simulink model "Block_PI_regulator"  (R2022a)
settings: Solver=ode23tb  StartTime=0.0  StopTime=6  MaxStep=1e4  RelTol=1e-5
undefined symbols (not defined in the file): DiscIntNeverNeededParam, PI_reg
settings Model: Creator=админ  LastModifiedBy=админ

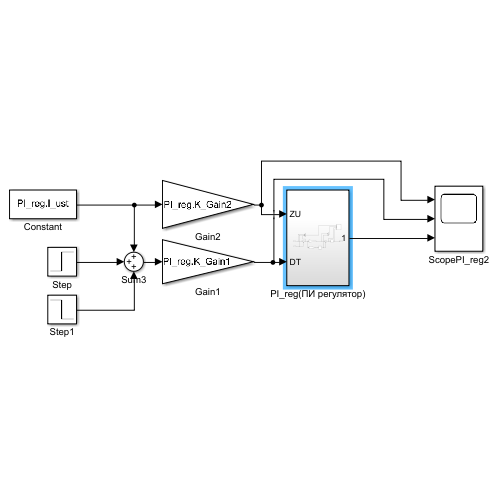
[thumbnail: Simulink's stored preview of the top-level diagram]
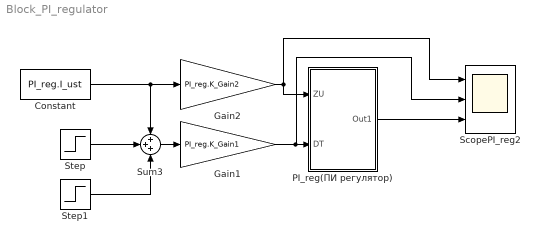
== system Block_PI_regulator ==
  Constant : Constant  Value=PI_reg.I_ust
  Gain1 : Gain  Gain=PI_reg.K_Gain1
  Gain2 : Gain  Gain=PI_reg.K_Gain2
  PI_reg(ПИ регулятор) : Subsystem
  ScopePI_reg2 : Scope  NumInputPorts=3
  Step : Step  Time=PI_reg.Step_time  After=PI_reg.Step_FinalValue  SampleTime=0
  Step1 : Step  Time=PI_reg.Step1_time  After=PI_reg.Step1_FinalValue  SampleTime=0
  Sum3 : Sum  Inputs=+++
  wires:
  Sum3/1 -> Gain1/1
  Gain1/1 -> ScopePI_reg2/2, PI_reg(ПИ регулятор)/2(DT)
  Gain2/1 -> PI_reg(ПИ регулятор)/1(ZU), ScopePI_reg2/1
  Constant/1 -> Sum3/1, Gain2/1
  Step/1 -> Sum3/2
  Step1/1 -> Sum3/3
  PI_reg(ПИ регулятор)/1(Out1) -> ScopePI_reg2/3

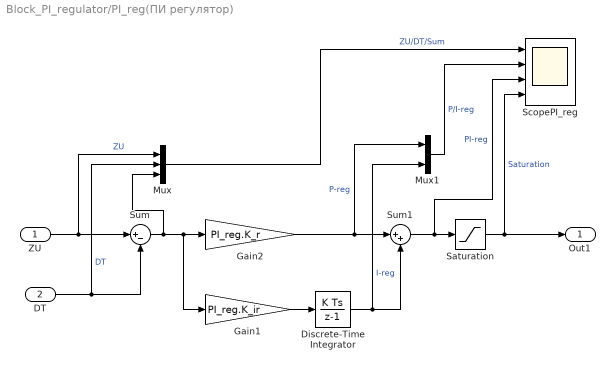
== system Block_PI_regulator/PI_reg(ПИ регулятор) ==
  ZU : Inport
  DT : Inport  Port=2
  Discrete-Time Integrator : DiscreteIntegrator  SampleTime=PI_reg.DTI_st  ICPrevOutput=DiscIntNeverNeededParam  ICPrevScaledInput=DiscIntNeverNeededParam
  Gain1 : Gain  Gain=PI_reg.K_ir
  Gain2 : Gain  Gain=PI_reg.K_r
  Mux : Mux  Inputs=3
  Mux1 : Mux  Inputs=2
  Saturation : Saturate  UpperLimit=PI_reg.StUp_limit  LowerLimit=PI_reg.StLow_limit
  ScopePI_reg : Scope  NumInputPorts=4
  Sum : Sum  Inputs=|+-
  Sum1 : Sum  Inputs=|++
  Out1 : Outport
  wires:
  Sum/1 -> Mux/3, Gain1/1, Gain2/1
  Discrete-Time Integrator/1 -> Mux1/2, Sum1/2  "I-reg"
  Gain2/1 -> Mux1/1, Sum1/1  "P-reg"
  ZU/1 -> Mux/1, Sum/1  "ZU"
  Gain1/1 -> Discrete-Time Integrator/1
  Saturation/1 -> Out1/1, ScopePI_reg/4  "Saturation"
  Sum1/1 -> ScopePI_reg/3, Saturation/1  "PI-reg"
  DT/1 -> Mux/2, Sum/2  "DT"
  Mux/1 -> ScopePI_reg/1  "ZU/DT/Sum"
  Mux1/1 -> ScopePI_reg/2  "P/I-reg"
